simulink model "Traffic_Light"  (R2016a)
settings: Solver=FixedStepDiscrete  StartTime=0.0  StopTime=10.0  FixedStep=0.1  RelTol=1e-3
model workspace (MAT data in the model file):
  cs : Simulink.ConfigSet (value not decoded)
settings Model: Creator=LEGION  LastModifiedBy=LEGION
settings SolverCC: AutoInsertRateTranBlk=on
settings DataIOCC: LimitDataPoints=on
settings DebuggingCC: AllowSymbolicDim=off
settings ConfigComp: CovModelRefEnable=Off  CovSFcnEnable=off

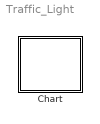
== system Traffic_Light ==
  Chart : Stateflow chart  TreatAsAtomicUnit=on

== stateflow chart Traffic_Light/Chart ==
  state Stop
  state PrepareToStop
  state GO
  (default) -> Stop
  PrepareToStop -> GO : [after(3,tick)]
  Stop -> PrepareToStop : [after(3,tick)]
  GO -> Stop : [after(3,tick)]
